simulink model "DPGandLQRsimOnlyIdentH"  (R2025b)
settings: Solver=VariableStepAuto  StartTime=0.0  StopTime=60000  FixedStep=1e-3  MaxStep=1e-3  RelTol=1e-3
values from neighbouring files (symbols this model uses):
  A = [1.0000    0.0099 ... (first row only)    [DPGandLQRIdentHandK.m]    (also in DPGandLQR_usingDlfevel.m = [1.0000, 0.0099; DPGandLQRsimOnlyIdentH.m)
  B = [4.9503e-05 ... (first row only)    [DPGandLQRIdentHandK.m]    (also in DPGandLQR_usingDlfevel.m; DPGandLQRsimOnlyIdentH.m)
  C = eye(size(A))    [DPGandLQRIdentHandK.m]    (also in DPGandLQRsimOnlyIdentH.m)
  H_critic = (H_critic + H_critic') / 2    [DPGandLQRIdentHandK.m]    (also in DPGandLQR_usingDlfevel.m = 0.5 * (H_critic + H_critic'); DPGandLQRsimOnlyIdentH.m)
  Herror = [1 1 1;1  1 1;1 1 1]*20    [DPGandLQRIdentHandK.m]    (also in DPGandLQRsimOnlyIdentH.m)
undefined symbols (not defined in the file or in its folder): K_lqr, magnitude
libraries: simulink x1
settings Model: PacingRate=3000  Creator=17547  LastModifiedBy=17547

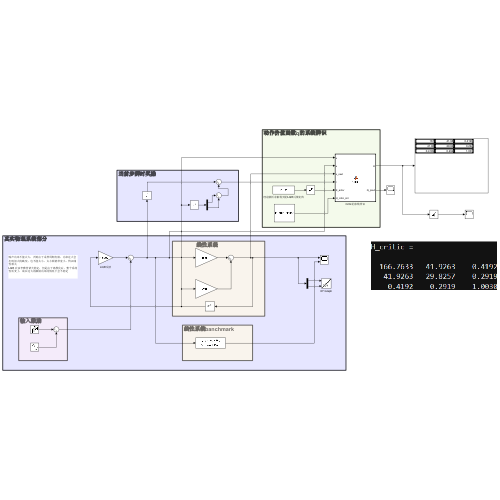
[thumbnail: Simulink's stored preview of the top-level diagram]
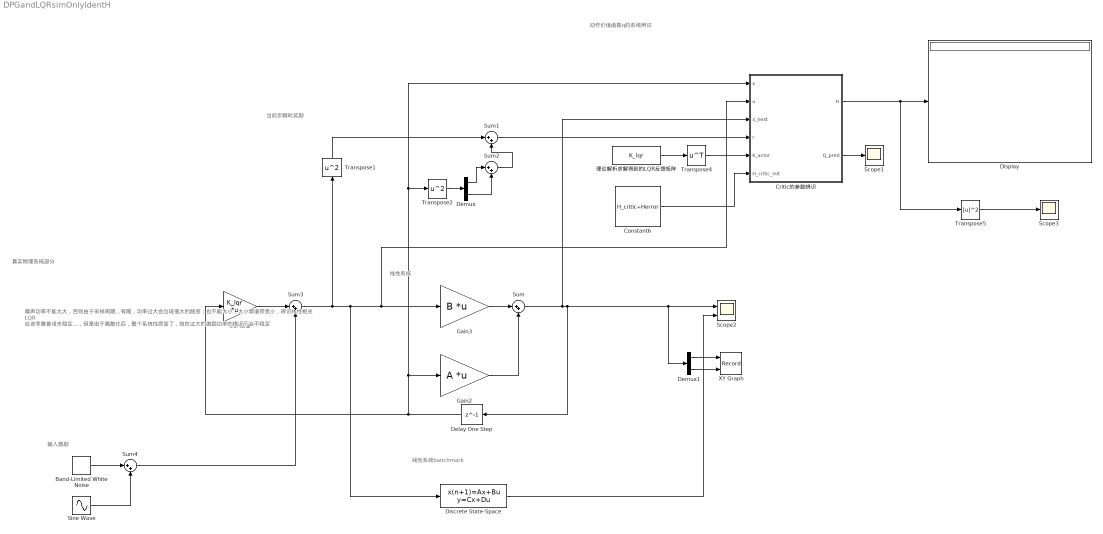
== system DPGandLQRsimOnlyIdentH ==
  note: 当前步瞬时奖励
  note: 线性系统banchmark
  note: 线性系统
  note: 输入激励
  note: 真实物理系统部分
  note: 噪声功率不能太大，否则由于采样周期有限，功率过大会出现很大的跳变；也不能太小，太小频谱带宽小，辨识线性相关
      | LQR 应该李雅普诺夫稳定，但是由于离散化后，整个系统性质变了，故在过大的激励功率的情况下会不稳定
  note: 动作价值函数q的系统辨识
  Band-Limited White Noise : simulink/Sources/Band-Limited White Noise  Cov=[0.004]  Ts=0.01  seed=[23341]
  Constant6 : Constant  Value=H_critic+Herror
  Critic的参数辨识 : MATLAB Function  TreatAsAtomicUnit=on
  Delay One Step : Delay  DelayLength=1
  Demux : Demux  Outputs=2
  Demux1 : Demux  Outputs=2
  Discrete State-Space : DiscreteStateSpace  A=A  B=B  C=C  D=zeros(size(B))  SampleTime=-1
  Display : Display
  Gain2 : Gain  Gain=A  Multiplication=Matrix(K*u)
  Gain3 : Gain  Gain=B  Multiplication=Matrix(K*u)
  LQR反馈 : Gain  Gain=K_lqr  Multiplication=Matrix(K*u) (u vector)
  Scope1 : Scope
      settings: ActiveDisplayYMinimum=-30.0192365044006  ActiveDisplayYMaximum=76.966685415106809  DataLoggingVariableName=ScopeData2
  Scope2 : Scope  NumInputPorts=2
      settings: ActiveDisplayYMinimum=-0.043537981572630356  ActiveDisplayYMaximum=-0.038024155226569774
  Scope3 : Scope
      settings: ActiveDisplayYMinimum=-4360.06615637184  ActiveDisplayYMaximum=39240.595408790767  DataLoggingVariableName=ScopeData3
  Sine Wave : Sin  Amplitude=2  Frequency=2  SampleTime=0
  Sum{,1..4} (5 alike) : Sum  Inputs=|++
  Transpose1 : Math  Operator=square
  Transpose2 : Math  Operator=square
  Transpose4 : Math  Operator=transpose
  Transpose5 : Math  Operator=magnitude^2
  XY Graph : Record  NumPorts=2.0  FileSettingsInternal="{\"entries\":[{\"content\":{\"excelSettings\":{\"content\":{},\"type\":\"Streamout.ExcelSettings\"},\"parquetSettings\":{\"content\":{},\"type\":\"Streamout.ParquetSettings\"}},\"type\":\"Streamout.FileSettingStorage\",\"uuid\":\"\"}],\"packageUris\":[\"http:\\/\\/schema.mathworks.com\\/mf0\\/streamout_blocks\\/R2020a\"],\"version\":\"1.0\"}"  FrameSettings=[0, 0]  Layout=[1 1]  SignalsInternal="{\"entries\":[{\"content\":{\"signals\":[{\"content\":{\"blockPath\":[],\"dimensions\":[1],\"domain\":\"\",\"lineColor\":\"#a2142f\",\"plots\":[ 1 ],\"port\":1,\"sid\":[\"\"],\"signalID\":1,\"signalName\":\"Demux1:1\"},\"type\":\"RecordBlkView.Signal\",\"uuid\":\"\"},{\"content\":{\"blockPath\":[],\"dimensions\":[1],\"domain\":\"\",\"lineColor\":\"#139fff\",\"plots\":[ 1 ],\"port\":2,\"sid\":[\"\"],\"signalID\":2,\"signalName\":\"Demux1:2\"},\"type\":\"RecordBlkView.Signal\",\"uuid\":\"\"}]},\"type\":\"RecordBlkView.InputSignals\",\"uuid\":\"\"}],\"packageUris\":[\"http:\\/\\/schema.mathworks.com\\/mf0\\/streamout_blocks\\/R2020a\"],\"version\":\"1.0\"}"  VisualizationBindings="{\"xyplotplugin\":{\"info\":[{\"series\":[{\"bindingParametersList\":[{\"parameter\":\"X-Axis\",\"signalID\":1,\"signalName\":\"Demux1:1\"},{\"parameter\":\"Y-Axis\",\"signalID\":2,\"signalName\":\"Demux1:2\"},{\"parameter\":\"X-Axis\",\"signalID\":1,\"signalName\":\"Demux1:1\"},{\"parameter\":\"Y-Axis\",\"signalID\":2,\"signalName\":\"Demux1:2\"},{\"parameter\":\"X-Axis\",\"signalID\":1,\"signalName\":\"Demux1:1\"},{\"parameter\":\"Y-Axis\",\"signalID\":2,\"signalName\":\"Demux1:2\"},{\"parameter\":\"X-Axis\",\"signalID\":1,\"signalName\":\"Demux1:1\"},{\"parameter\":\"Y-Axis\",\"signalID\":2,\"signalName\":\"Demux1:2\"}],\"seriesID\":0}],\"subplotID\":1}]}}"  CompatibilityTag=XY
  理论解析求解得到的LQR反馈矩阵 : Constant  Value=K_lqr
  wires:
  Constant6/1 -> Critic的参数辨识/6(H_critic_init)
  Gain3/1 -> Sum/1
  Gain2/1 -> Sum/2
  Delay One Step/1 -> Gain2/1, Transpose2/1, Critic的参数辨识/1(x), LQR反馈/1
  Sum/1 -> Demux1/1, Scope2/1, Delay One Step/1, Critic的参数辨识/3(x_next)
  Sum3/1 -> Discrete State-Space/1, Gain3/1, Critic的参数辨识/2(u), Transpose1/1
  Sum1/1 -> Critic的参数辨识/4(r)
  Transpose1/1 -> Sum1/1
  Transpose2/1 -> Demux/1
  理论解析求解得到的LQR反馈矩阵/1 -> Transpose4/1
  Demux/2 -> Sum2/2
  Demux/1 -> Sum2/1
  Sum2/1 -> Sum1/2
  Transpose4/1 -> Critic的参数辨识/5(K_actor)
  Discrete State-Space/1 -> Scope2/2
  LQR反馈/1 -> Sum3/1
  Critic的参数辨识/2(Q_pred) -> Scope1/1
  Critic的参数辨识/1(H) -> Transpose5/1, Display/1
  Transpose5/1 -> Scope3/1
  Band-Limited White Noise/1 -> Sum4/1
  Sum4/1 -> Sum3/2
  Sine Wave/1 -> Sum4/2
  Demux1/1 -> XY Graph/1
  Demux1/2 -> XY Graph/2

== matlab function DPGandLQRsimOnlyIdentH/Critic的参数辨识 ==
  data: x input; u input; x_next input; r input; K_actor input; H output; H_critic_init input; Q_pred output
function [H,Q_pred] = Critic(x, u, x_next, r, K_actor, H_critic_init)
 
    persistent H_critic  % 生命周期持续到仿真结束
    if isempty(H_critic)
        H_critic = H_critic_init;  % 用输入端口设置初值
    end

    gamma = 1;
    alpha_critic = 0.005;
    % 更新 Critic (Policy Evaluation, TD-Learning) ---
    
    z = [x; u];
    
    % 目标策略 (Target Policy): 评估当前 Actor 的纯策略 (无噪声)
    u_next = -K_actor * x_next; 
    z_next = [x_next; u_next];
    
    % 计算 TD 误差: 预测值 vs 目标值 (半梯度法，不对目标求导)
    Q_pred = z' * H_critic * z;
    Q_target = r + gamma * (z_next' * H_critic * z_next);
    delta = Q_pred - Q_target;
    
    %  Critic 梯度: \nabla_H Loss = delta * z * z'    % deepseek J = v'Hv  对H求梯度  等于什么
    TDerrwithG = delta * (z * z');

    % 梯度下降更新 H，并强制对称化
    H_critic = H_critic - alpha_critic * (TDerrwithG);
    H_critic = (H_critic + H_critic') / 2; 
    H = H_critic;
end
